simulink model "test_commutator"  (Simulink 6.2)
settings: Solver=ode45  StartTime=0.0  StopTime=50.0  RelTol=1e-3
libraries: xbsIndex_r3 x14, simulink x1
settings Model: LastModifiedBy=mdexter
settings DebuggingCC: SolverPrmCheckMsg=warning

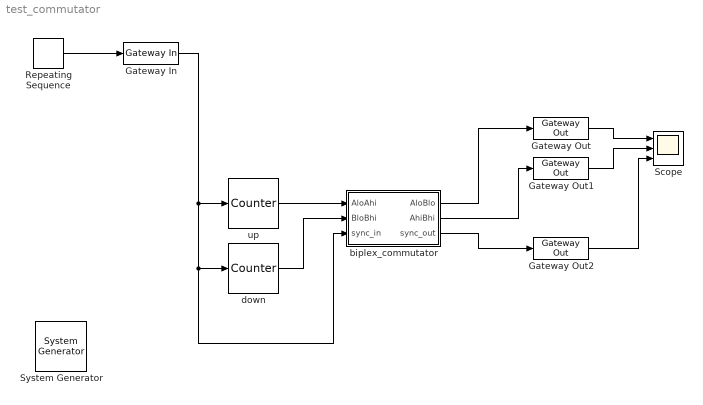
== system test_commutator ==
  " System Generator" : xbsIndex_r3/ System Generator  Tag=genX  xilinxfamily=Virtex2  part=xc2v1000  speed=-4  package=bg575  synthesis_tool=XST  directory=./netlist.tmp  testbench=off  simulink_period=1  sysclk_period=100  incr_netlist=off  trim_vbits=Everywhere in SubSystem  dbl_ovrd=According to Block Masks  core_generation=According to Block Masks  run_coregen=off  deprecated_control=off  eval_field=0
      settings: AttributesFormatString=System\nGenerator
  Gateway In : xbsIndex_r3/Gateway In  arith_type=Boolean  n_bits=8  bin_pt=6  quantization=Truncate  overflow=Wrap  period=1  timing_constraint=None  locs_specified=off  LOCs={}  needs_fixed_name=off  dbl_ovrd=off  show_param=off
      settings: xl_area=[0, 0, 0, 0, 0, 0, 0]
  Gateway Out : xbsIndex_r3/Gateway Out  output_type=Double  nbits=8  bin_pt=6  arith_type=Boolean  quantization=Truncate  overflow=Wrap  hdl_port=on  timing_constraint=None  locs_specified=off  LOCs={}  needs_fixed_name=off  show_param=off
      settings: xl_area=[0, 0, 0, 0, 0, 0, 0]
  Gateway Out1 : xbsIndex_r3/Gateway Out  output_type=Double  nbits=8  bin_pt=6  arith_type=Boolean  quantization=Truncate  overflow=Wrap  hdl_port=on  timing_constraint=None  locs_specified=off  LOCs={}  needs_fixed_name=off  show_param=off
      settings: xl_area=[0, 0, 0, 0, 0, 0, 0]
  Gateway Out2 : xbsIndex_r3/Gateway Out  output_type=Double  nbits=8  bin_pt=6  arith_type=Boolean  quantization=Truncate  overflow=Wrap  hdl_port=on  timing_constraint=None  locs_specified=off  LOCs={}  needs_fixed_name=off  show_param=off
      settings: xl_area=[0, 0, 0, 0, 0, 0, 0]
  Repeating Sequence : simulink/Sources/Repeating Sequence  rep_seq_t=[0:32]  rep_seq_y=[1 zeros(1,31) 1]
  Scope : Scope  NumInputPorts=3
      settings: YMin=-5~-5~-5  YMax=5~5~5
  biplex_commutator : Subsystem  mask(Biplex Commutator){log2_size=2, n_bits=2, use_bram=off}
      mask prompts: log2_size "Log2 Block Size"; n_bits "Bit Width"; use_bram "Use BRAM"
      mask help: The biplex commutator commutes the first half of the BloBhi input "block" with the last half of the AloAhi input "block". A "block" is 2^log2_size consecutive samples (i.e. always a power of 2). sync_in precedes the first data input sample by one clock cycle. Overall latency from sync_in to sync_out is 2^(log2_size-1)+1.
      mask init:
      | biplex_commutator_init(gcb, ...
      |     log2_size, ...
      |     n_bits, ...
      |     use_bram);
      settings: AttributesFormatString=|
      | size = 4
      | delay slr
      mask Help:
      | <pre>
      | Description::
      | 
      | The biplex commutator commutes the first half of the BloBhi input "block"  with the last half
      | of the AloAhi input "block".  A "block" is 2^log2_size consecutive samples (i.e. always a
      | power of 2).
      | 
      | sync_in precedes the first data input sample by one clock cycle.
      | sync_out precedes the corresponding output sample by one clock cycle.
      | Overall latency from sync_in to sync_out is 2^(N-1)+1.
      | 
      | Mask Parameters::
      | 
      | Log 2 Block Size (log2_size): The base-2 logarithm of the length of one complete input block.
      | This MUST be an integer because the current implementation requires that
      | the input block size MUST be a power of 2.  (aka "N")
      | 
      | Bit Width (n_bits): Specifies the width of the real/imaginary components.
      | Width of each component is assumed equal.
      | 
      | Use BRAM (use_bram): Check this checkbox to implement the internal delays using BRAM.
      | If unchecked, the internal delays will be implemented using SLR16 elements.
      | </pre>
  down : xbsIndex_r3/Counter  cnt_type=Free Running  n_bits=4  bin_pt=0  arith_type=Unsigned  start_count=15  cnt_to=Inf  cnt_by_val=1  operation=Down  explicit_period=off  period=1  load_pin=off  rst=on  en=off  dbl_ovrd=off  show_param=off  use_rpm=on  gen_core=off
      settings: xl_area=[0, 0, 0, 0, 0, 0, 0]
  up : xbsIndex_r3/Counter  cnt_type=Free Running  n_bits=4  bin_pt=0  arith_type=Unsigned  start_count=0  cnt_to=Inf  cnt_by_val=1  operation=Up  explicit_period=off  period=1  load_pin=off  rst=on  en=off  dbl_ovrd=off  show_param=off  use_rpm=on  gen_core=off
      settings: xl_area=[0, 0, 0, 0, 0, 0, 0]
  wires:
  Gateway Out/1 -> Scope/1
  Gateway Out1/1 -> Scope/2
  Repeating Sequence/1 -> Gateway In/1
  Gateway In/1 -> up/1, down/1, biplex_commutator/3(sync_in)
  up/1 -> biplex_commutator/1(AloAhi)
  biplex_commutator/1(AloBlo) -> Gateway Out/1
  down/1 -> biplex_commutator/2(BloBhi)
  biplex_commutator/2(AhiBhi) -> Gateway Out1/1
  biplex_commutator/3(sync_out) -> Gateway Out2/1
  Gateway Out2/1 -> Scope/3

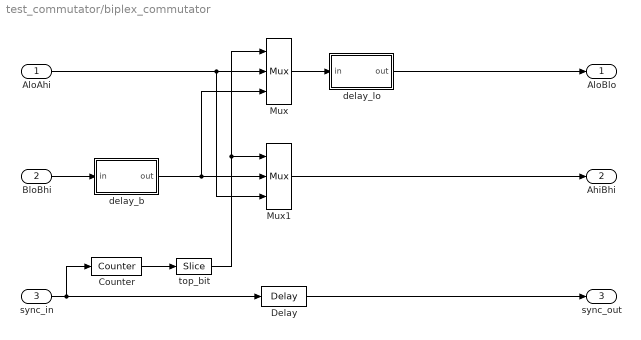
== system test_commutator/biplex_commutator ==
  AloAhi : Inport  Port=1  LatchInput=off
  BloBhi : Inport  Port=2  LatchInput=off
  sync_in : Inport  Port=3  LatchInput=off
  Counter : xbsIndex_r3/Counter  cnt_type=Free Running  n_bits=2  bin_pt=0  arith_type=Unsigned  start_count=0  cnt_to=Inf  cnt_by_val=1  operation=Up  explicit_period=off  period=1  load_pin=off  rst=on  en=off  dbl_ovrd=off  show_param=off  use_rpm=on  gen_core=off
      settings: xl_area=[0, 0, 0, 0, 0, 0, 0]
  Delay : xbsIndex_r3/Delay  latency=3  reg_retiming=off  explicit_period=off  period=1  en=off  accept_only_valid=off  init_zero=on  dbl_ovrd=off  show_param=off
      settings: xl_area=[0, 0, 0, 0, 0, 0, 0]
  Mux : xbsIndex_r3/Mux  inputs=2  precision=Full  arith_type="Signed  (2's comp)"  n_bits=8  bin_pt=2  quantization=Truncate  overflow=Wrap  latency=1  explicit_period=off  period=1  en=off  dbl_ovrd=off  show_param=off  mux_type=off  use_rpm=off  gen_core=off
      settings: xl_area=[0, 0, 0, 0, 0, 0, 0]
  Mux1 : xbsIndex_r3/Mux  inputs=2  precision=Full  arith_type="Signed  (2's comp)"  n_bits=8  bin_pt=2  quantization=Truncate  overflow=Wrap  latency=1  explicit_period=off  period=1  en=off  dbl_ovrd=off  show_param=on  mux_type=off  use_rpm=off  gen_core=off
      settings: xl_area=[0, 0, 0, 0, 0, 0, 0]
  delay_b : Subsystem  mask(SLR16 Delay){delay_depth=2}
      mask prompts: delay_depth "Delay Depth"
      mask help: A delay block that uses SLR16 elements for its storage.
      settings: AttributesFormatString=slr depth = 2
      mask Help:
      | <pre>
      | Description::
      | 
      | A delay block that uses SLR16 elements for its storage.
      | 
      | Mask Parameters::
      | 
      | Delay Depth (delay_depth): The length of the delay.
      | </pre>
  delay_lo : Subsystem  mask(SLR16 Delay){delay_depth=2}
      mask prompts: delay_depth "Delay Depth"
      mask help: A delay block that uses SLR16 elements for its storage.
      settings: AttributesFormatString=slr depth = 2
      mask Help:
      | <pre>
      | Description::
      | 
      | A delay block that uses SLR16 elements for its storage.
      | 
      | Mask Parameters::
      | 
      | Delay Depth (delay_depth): The length of the delay.
      | </pre>
  top_bit : xbsIndex_r3/Slice  mode=Upper Bit Location + Width  nbits=1  bit1=0  base1=MSB of Input  bit0=0  base0=LSB of Input  boolean_output=off  explicit_period=off  period=1  dbl_ovrd=off
  AloBlo : Outport
  AhiBhi : Outport  Port=2
  sync_out : Outport  Port=3
  wires:
  Delay/1 -> sync_out/1
  delay_lo/1(out) -> AloBlo/1
  Mux/1 -> delay_lo/1(in)
  delay_b/1(out) -> Mux/3, Mux1/2
  BloBhi/1 -> delay_b/1(in)
  Mux1/1 -> AhiBhi/1
  AloAhi/1 -> Mux1/3, Mux/2
  top_bit/1 -> Mux/1, Mux1/1
  Counter/1 -> top_bit/1
  sync_in/1 -> Delay/1, Counter/1

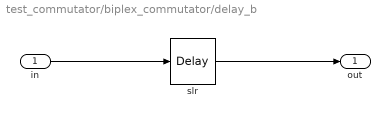
== system test_commutator/biplex_commutator/delay_b ==
  in : Inport  Port=1  LatchInput=off
  slr : xbsIndex_r3/Delay  latency=2  reg_retiming=off  explicit_period=off  period=1  en=off  accept_only_valid=off  init_zero=on  dbl_ovrd=off  show_param=off
      settings: xl_area=[0, 0, 0, 0, 0, 0, 0]
  out : Outport
  wires:
  slr/1 -> out/1
  in/1 -> slr/1

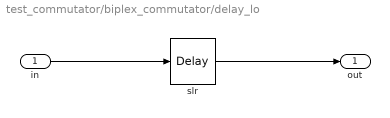
== system test_commutator/biplex_commutator/delay_lo ==
  in : Inport  Port=1  LatchInput=off
  slr : xbsIndex_r3/Delay  latency=2  reg_retiming=off  explicit_period=off  period=1  en=off  accept_only_valid=off  init_zero=on  dbl_ovrd=off  show_param=off
      settings: xl_area=[0, 0, 0, 0, 0, 0, 0]
  out : Outport
  wires:
  slr/1 -> out/1
  in/1 -> slr/1
